simulink model "duplointegradorSIN"  (Simulink 7.7)
settings: Solver=ode3  StartTime=0.0  StopTime=100  FixedStep=0.01  RelTol=1e-3
libraries: simulink x1
settings Model: Creator=josenaldeoliveira  LastModifiedBy=josenaldeoliveira

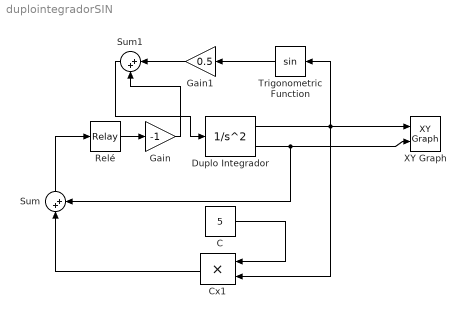
== system duplointegradorSIN ==
  C : Constant  Value=5
  Cx1 : Product  RndMeth=Zero
  Duplo Integrador : SecondOrderIntegrator  ICX=0.5  StateNameX='X1'  ICDXDT=0.5  StateNameDXDT='X2'
  Gain : Gain  Gain=-1  SampleTime=0.01
  Gain1 : Gain  Gain=0.5  SampleTime=0.01
  Relé : Relay  OnSwitchValue=0.00000001  OffSwitchValue=-0.0000001  OffOutputValue=-1  SampleTime=0.01
  Sum : Sum  Inputs=|++
  Sum1 : Sum  Inputs=|++
  Trigonometric Function : Trigonometry
  XY Graph : simulink/Sinks/XY Graph  SystemSampleTime=-1  xmin=-1  xmax=1  ymin=-1  ymax=1  st=0.01
  wires:
  C/1 -> Cx1/1
  Duplo Integrador/1 -> Cx1/2, XY Graph/1, Trigonometric Function/1
  Duplo Integrador/2 -> Sum/2, XY Graph/2
  Cx1/1 -> Sum/1
  Sum/1 -> Relé/1
  Relé/1 -> Gain/1
  Trigonometric Function/1 -> Gain1/1
  Gain1/1 -> Sum1/1
  Gain/1 -> Sum1/2
  Sum1/1 -> Duplo Integrador/1
